simulink model "fcn"  (R2018a)
settings: Solver=VariableStepAuto  StartTime=0.0  StopTime=inf  RelTol=1e-3
undefined symbols (not defined in the file or in its folder): serial
libraries: instrumentlib x3, etargetslib x1
settings Model: Creator=Benjamin Nicolas  LastModifiedBy=Benjamin Nicolas

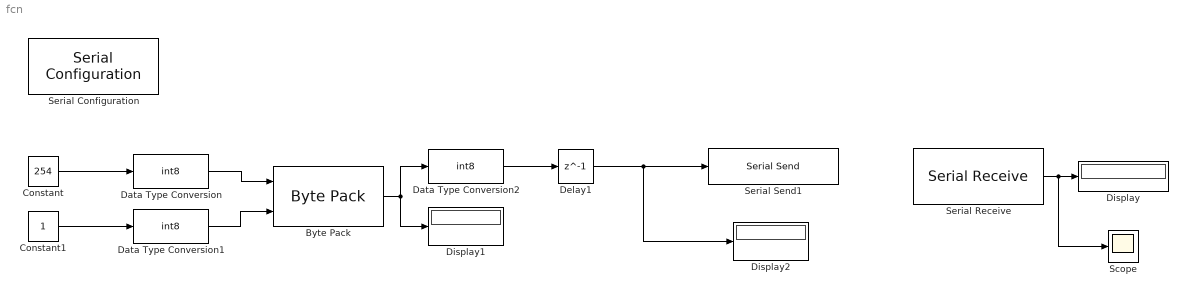
== system fcn ==
  Byte Pack : etargetslib/Byte Pack  datatypes={'int8','int8'}  byteAlign=1
  Constant : Constant  Value=254
  Constant1 : Constant
  Data Type Conversion : DataTypeConversion  OutDataTypeStr=int8
  Data Type Conversion1 : DataTypeConversion  OutDataTypeStr=int8
  Data Type Conversion2 : DataTypeConversion  OutDataTypeStr=int8
  Delay1 : Delay  DelayLength=1  InitialCondition=0  SampleTime=0.02
  Display : Display
  Display1 : Display
  Display2 : Display
  Scope : Scope
  Serial Configuration : instrumentlib/Serial Configuration  Priority=-200000  ComPortMenu=COM4  ComPort=COM4  ObjConstructor=serial('COM4');  BaudRate=128000  DataBits=8  Parity=none  StopBits=1  FlowControl=none  Timeout=10  ByteOrder=LittleEndian
  Serial Receive : instrumentlib/Serial Receive  ComPortMenu=COM4  ComPort=COM4  ObjConstructor=serial('COM4');  Terminator=<none>  DataSize=[1 1]  DataType=uint8  EnableBlockingMode=on  ActionDataUnavailable=Output last received value  CustomValue=0  SampleTime=0.02
  Serial Send1 : instrumentlib/Serial Send  ComPortMenu=COM4  ComPort=COM4  ObjConstructor=serial('COM4');  Terminator=<none>  EnableBlockingMode=off
  wires:
  Constant/1 -> Data Type Conversion/1
  Constant1/1 -> Data Type Conversion1/1
  Data Type Conversion/1 -> Byte Pack/1
  Byte Pack/1 -> Data Type Conversion2/1, Display1/1
  Data Type Conversion1/1 -> Byte Pack/2
  Data Type Conversion2/1 -> Delay1/1
  Delay1/1 -> Display2/1, Serial Send1/1
  Serial Receive/1 -> Scope/1, Display/1
